simulink model "HeatSourceAWHPModel"  (R2024a)
settings: Solver=VariableStepAuto  StartTime=0.0  StopTime=60  RelTol=1e-3
libraries: fl_lib x7, nesl_utility x4
settings Model: Creator=vikrants  LastModifiedBy=vikrants

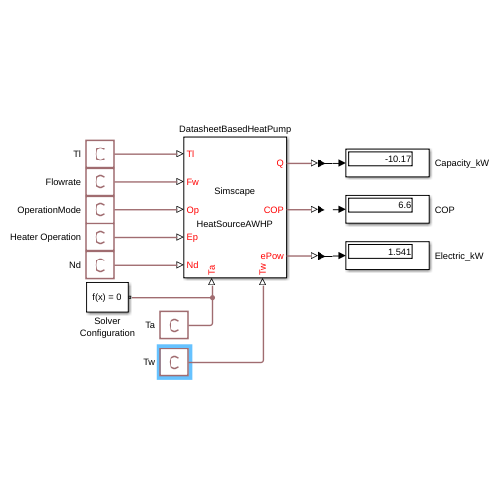
[thumbnail: Simulink's stored preview of the top-level diagram]
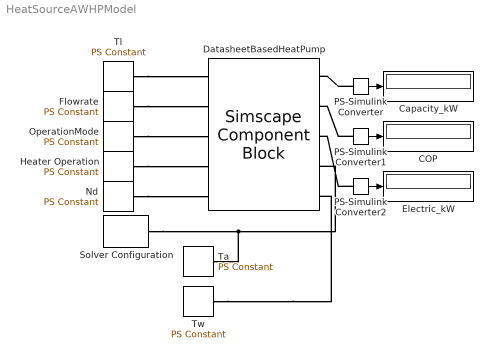
== system HeatSourceAWHPModel ==
  COP : Display
  Capacity_kW : Display
  DatasheetBasedHeatPump : SimscapeComponentBlock  SourceFile=HeatSourceAWHP  ComponentPath=HeatSourceAWHP  ComponentVariants="[\"HeatSourceAWHP\"]"  ComponentVariantNames="[\"HeatSourceAWHP\"]"  ClassName=HeatSourceAWHP  SchemaVersion=1  nominalCapacityA=10.17 kW  seasonalCOPvalA=4.86  nominalCapacityB=10.12 kW  seasonalCOPvalB=3.7  nominalCapacityC=10.17 kW  seasonalCOPvalC=4.86  nominalCapacityD=10.12 kW  seasonalCOPvalD=3.7  nominalCapacityE=10.55 kW  seasonalCOPvalE=4.13  nominalCapacityF=6.9 kW  seasonalCOPvalF=2.7  backupElecHeater=1 kW  wInletOpRangeUpp=330 K  wInletOpRangeLow=278 K  airTemperatureVector=273 + [-2, -2, 7, 7, 35, 35]  waterTemperatureVector=273 + [55, 65, 35, 45, 18, 7]  waterSpHeat=4186 J/(K*kg)  smallPower=1e-3 W  maxCOP_specify=off  maxCOP_priority=None  maxCOP=8  maxCOP_nominal_specify=off  maxCOP_nominal_value=1  maxCOP_nominal_unit=1
      settings: CopyFcn=simscape.engine.sli.internal.componentblockcallback(gcbh,'COPY')  PreCopyFcn=simscape.engine.sli.internal.componentblockcallback(gcbh,'PRECOPY')  PreDeleteFcn=simscape.engine.sli.internal.componentblockcallback(gcbh,'PREDELETE')  InternalSimscapePortConfiguration="{\"Bottom\":[{\"id\":\"Ta\",\"label\":\"Ta\",\"type\":\"input\"},{\"id\":\"Tw\",\"label\":\"Tw\",\"type\":\"input\"}],\"Left\":[{\"id\":\"Tl\",\"label\":\"Tl\",\"type\":\"input\"},{\"id\":\"Fw\",\"label\":\"Fw\",\"type\":\"input\"},{\"id\":\"Op\",\"label\":\"Op\",\"type\":\"input\"},{\"id\":\"Ep\",\"label\":\"Ep\",\"type\":\"input\"},{\"id\":\"Nd\",\"label\":\"Nd\",\"type\":\"input\"}],\"Right\":[{\"id\":\"calcCap\",\"label\":\"Q\",\"type\":\"output\"},{\"id\":\"calcCOP\",\"label\":\"COP\",\"type\":\"output\"},{\"id\":\"ePower\",\"label\":\"ePow\",\"type\":\"output\"}],\"Top\":[]}"
      mask Type: HeatSourceAWHP
  Electric_kW : Display
  Flowrate : fl_lib/Physical Signals/Sources/PS Constant  constant=0.5 kg/s
  Heater Operation : fl_lib/Physical Signals/Sources/PS Constant  constant=0
  Nd : fl_lib/Physical Signals/Sources/PS Constant  constant=1
  OperationMode : fl_lib/Physical Signals/Sources/PS Constant  constant=-1
  PS-Simulink Converter : nesl_utility/PS-Simulink Converter  PhysicalDomain=network_engine_domain  SubClassName=ps_output  LeftPortType=input  RightPortType=output  PseudoPeriodic=off  Frequencies=[]  VectorFormat=inherit  Unit=inherit  AffineConversion=off
  PS-Simulink Converter1 : nesl_utility/PS-Simulink Converter  PhysicalDomain=network_engine_domain  SubClassName=ps_output  LeftPortType=input  RightPortType=output  PseudoPeriodic=off  Frequencies=[]  VectorFormat=inherit  Unit=inherit  AffineConversion=off
  PS-Simulink Converter2 : nesl_utility/PS-Simulink Converter  PhysicalDomain=network_engine_domain  SubClassName=ps_output  LeftPortType=input  RightPortType=output  PseudoPeriodic=off  Frequencies=[]  VectorFormat=inherit  Unit=inherit  AffineConversion=off
  Solver Configuration : nesl_utility/Solver Configuration  PhysicalDomain=network_engine_domain  SubClassName=solver  LeftPortType=input  RightPortType=generic  Tones=[]  Harmonics=[]  SimulateNoise=off  Profile=off  UseLocalSampling=off  EnableSwitchedLinearOptims=on  FrequencyDomain=off  UseCCode=off  RelTol=0.001  AbsTol=1e-06  MinStep=1e-09  ToWorkspace=off  RevertToSquareIcSolve=off  NumHomotopyIterations=100  PhasorMode=off  PhasorModeNumHarmonics=1  ConsistencySolver=NEWTON_XTOL_AFTER_FTOL  IndexReductionMethod=DerivativeReplacement  DoDC=off  ResidualTolerance=1e-09  ConsistencyTolSource=GLOBAL  ConsistencyAbsTol=0.001  ConsistencyRelTol=0.001  ConsistencyTolFactor=0.001  UseLocalSolver=off  LocalSolverChoice=NE_BACKWARD_EULER_ADVANCER  ResolveIndetEquations=on  FunctionEvalNumThread=1  LocalSolverSampleTime=0.001  DoFixedCost=off  MaxNonlinIter=3  MaxModeIter=2  ComputeImpulses=off  ImpulseIterations=2  LinearAlgebra=auto  LinearAlgebraNumThread=0  EquationFormulation=NE_TIME_EF  DelaysMemoryBudget=1024  AutomaticFiltering=on  FilteringTimeConstant=0.001  PartitionStorageMethod=AS_NEEDED  PartitionMemoryBudget=1024  PartitionMethod=ROBUST  MultibodyUseLocalSolver=off  MultibodyLocalSolverChoice=ODE1  MultibodyLocalSolverSampleTime=0.001
  Ta : fl_lib/Physical Signals/Sources/PS Constant  constant=271 K
  Tl : fl_lib/Physical Signals/Sources/PS Constant  constant=311 K
  Tw : fl_lib/Physical Signals/Sources/PS Constant  constant=313 K
  wires:
  PS-Simulink Converter1/1 -> COP/1
  PS-Simulink Converter/1 -> Capacity_kW/1
  PS-Simulink Converter2/1 -> Electric_kW/1
  connections:
  Tw/RConn1 -- DatasheetBasedHeatPump/RConn5
  PS-Simulink Converter/LConn1 -- DatasheetBasedHeatPump/RConn1
  PS-Simulink Converter1/LConn1 -- DatasheetBasedHeatPump/RConn2
  PS-Simulink Converter2/LConn1 -- DatasheetBasedHeatPump/RConn3
  Ta/RConn1 -- Solver Configuration/RConn1 -- DatasheetBasedHeatPump/RConn4
  Nd/RConn1 -- DatasheetBasedHeatPump/LConn5
  Heater Operation/RConn1 -- DatasheetBasedHeatPump/LConn4
  OperationMode/RConn1 -- DatasheetBasedHeatPump/LConn3
  Flowrate/RConn1 -- DatasheetBasedHeatPump/LConn2
  Tl/RConn1 -- DatasheetBasedHeatPump/LConn1
